simulink subsystem "Subsystem"  (R2025b)
settings: Solver=VariableStepAuto  StartTime=0.0  StopTime=10.0  RelTol=1e-3
values from neighbouring files (symbols this model uses):
  b2_ext = x(5)    [f_dynamics.m]    (also in f_dynamics_Wo_DT.m = 96.1986389127)
  b2_ret = x(6)    [f_dynamics.m]    (also in f_dynamics_Wo_DT.m = 15.072)
  Q = double(Q)    [EKF_delay_compensated.m]    (also in NO_DT_EKF_delay_compensated.m)
undefined symbols (not defined in the file or in its folder): P, T_S, x_0
libraries: simulink x1
settings Model: Creator=Mohamed Reda  LastModifiedBy=Mohamed Reda

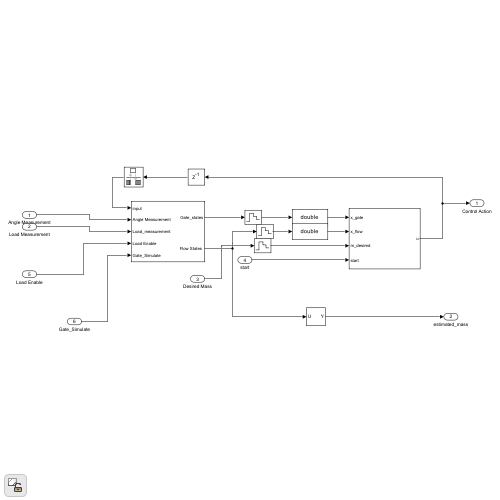
[thumbnail: Simulink's stored preview of the top-level diagram]
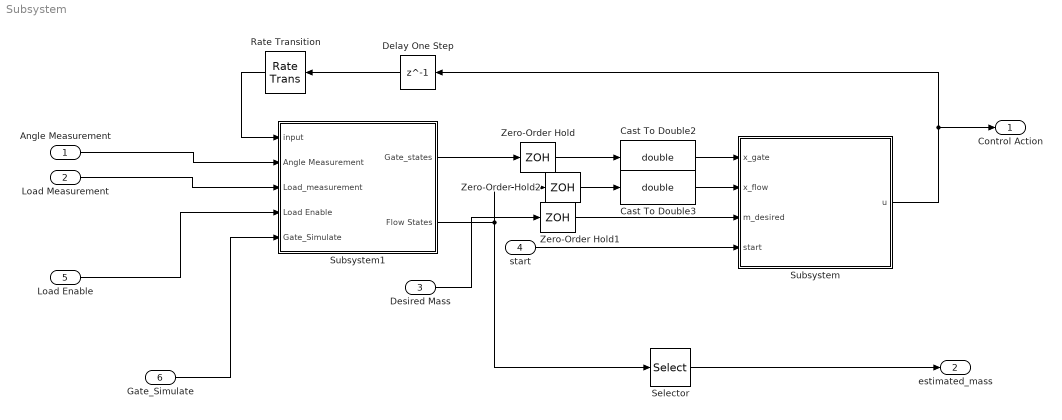
== system Subsystem ==
  Angle Measurement : Inport
  Load Measurement : Inport  Port=2
  Desired Mass : Inport  Port=3
  start : Inport  Port=4  SampleTime=5e-3
  Load Enable : Inport  Port=5
  Gate_Simulate : Inport  Port=6
  Cast To Double2 : DataTypeConversion  OutDataTypeStr=double  SaturateOnIntegerOverflow=off  RndMeth=Floor
  Cast To Double3 : DataTypeConversion  OutDataTypeStr=double  SaturateOnIntegerOverflow=off  RndMeth=Floor
  Delay One Step : Delay  DelayLength=1
  Rate Transition : RateTransition  OutPortSampleTime=2e-4
  Selector : Selector  InputPortWidth=9  IndexOptions=Index vector (dialog)  Indices=[2]  OutputSizes=1
  Subsystem : Subsystem
  Subsystem1 : Subsystem
  Zero-Order Hold : ZeroOrderHold  SampleTime=5e-3
  Zero-Order Hold1 : ZeroOrderHold  SampleTime=.5e-2
  Zero-Order Hold2 : ZeroOrderHold  SampleTime=5e-3
  Control Action : Outport
  estimated_mass : Outport  Port=2
  wires:
  Subsystem1/1(Gate_states) -> Zero-Order Hold/1
  Rate Transition/1 -> Subsystem1/1(input)
  Zero-Order Hold1/1 -> Subsystem/3(m_desired)
  Cast To Double3/1 -> Subsystem/2(x_flow)
  Delay One Step/1 -> Rate Transition/1
  Zero-Order Hold2/1 -> Cast To Double3/1
  Subsystem1/2("Flow States ") -> Selector/1, Zero-Order Hold2/1
  start/1 -> Subsystem/4(start)
  Cast To Double2/1 -> Subsystem/1(x_gate)
  Zero-Order Hold/1 -> Cast To Double2/1
  Selector/1 -> estimated_mass/1
  Subsystem/1(u) -> Control Action/1, Delay One Step/1
  Desired Mass/1 -> Zero-Order Hold1/1
  Angle Measurement/1 -> Subsystem1/2(Angle Measurement)
  Load Measurement/1 -> Subsystem1/3(Load_measurement)
  Load Enable/1 -> Subsystem1/4(Load Enable)
  Gate_Simulate/1 -> Subsystem1/5(Gate_Simulate)

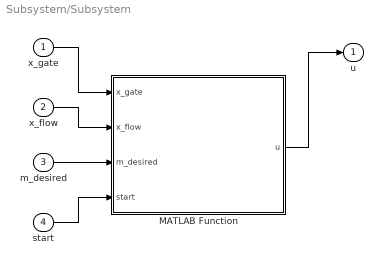
== system Subsystem/Subsystem ==
  x_gate : Inport  OutDataTypeStr=double  PortDimensions=7  SampleTime=[0.0050000000000000001,0]
  x_flow : Inport  Port=2  OutDataTypeStr=double  PortDimensions=9  SampleTime=[0.0050000000000000001,0]
  m_desired : Inport  Port=3  OutDataTypeStr=double  PortDimensions=1  SampleTime=[0.0050000000000000001,0]
  start : Inport  Port=4  OutDataTypeStr=double  PortDimensions=1  SampleTime=[0.0050000000000000001,0]
  MATLAB Function : MATLAB Function  TreatAsAtomicUnit=on
  u : Outport  OutDataTypeStr=double  PortDimensions=1  SampleTime=[0.0050000000000000001,0]
  wires:
  start/1 -> MATLAB Function/4(start)
  x_flow/1 -> MATLAB Function/2(x_flow)
  x_gate/1 -> MATLAB Function/1(x_gate)
  MATLAB Function/1(u) -> u/1
  m_desired/1 -> MATLAB Function/3(m_desired)

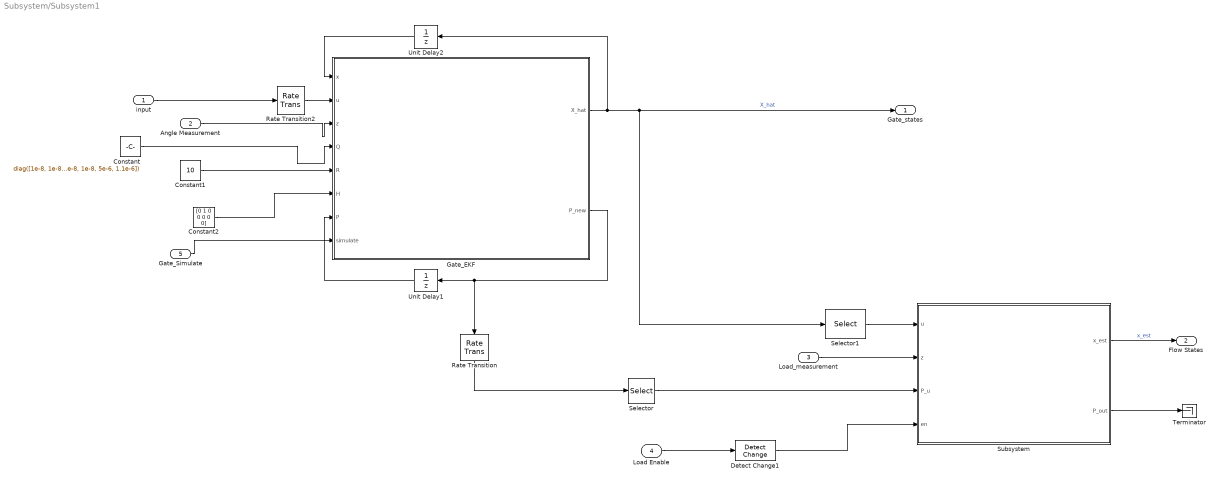
== system Subsystem/Subsystem1 ==
  input : Inport  OutDataTypeStr=double  PortDimensions=1  SampleTime=[0.00020000000000000001,0]
  Angle Measurement : Inport  Port=2  OutDataTypeStr=double  PortDimensions=1  SampleTime=[0.00020000000000000001,0]
  Load_measurement : Inport  Port=3  OutDataTypeStr=double  PortDimensions=1  SampleTime=[0.001,0]
  Load Enable : Inport  Port=4  OutDataTypeStr=boolean  PortDimensions=1  SampleTime=[0.001,0]
  Gate_Simulate : Inport  Port=5
  Constant : Constant  Value=diag([1e-8, 1e-8, 1e-8, 1e-8, 1e-8, 5e-6, 1.1e-6])
  Constant1 : Constant  Value=10
  Constant2 : Constant  Value=[0 1 0 0 0 0 0]
  Detect Change1 : simulink/Logic and Bit Operations/Detect Change  vinit=0  OutDataTypeStr=boolean
  Gate_EKF : MATLAB Function  TreatAsAtomicUnit=on
  Rate Transition : RateTransition
  Rate Transition2 : RateTransition
  Selector : Selector  NumberOfDimensions=2  InputPortWidth=7,7  IndexOptions=Index vector (dialog),Index vector (dialog)  Indices=1,1  OutputSizes=1,1
  Selector1 : Selector  InputPortWidth=7  IndexOptions=Index vector (dialog)  Indices=1  OutputSizes=1
  Subsystem : Subsystem
  Terminator : Terminator
  Unit Delay1 : UnitDelay  InitialCondition=diag([1e-6 1e-6 0.1 0.1 0.1 1e-6 1e-6])  SampleTime=-1  HasFrameUpgradeWarning=on
  Unit Delay2 : UnitDelay  InitialCondition=[deg2rad(0);0;9*101325;9*101325;101325;b2_ext;b2_ret]  SampleTime=-1  HasFrameUpgradeWarning=on
  Gate_states : Outport  OutDataTypeStr=double  PortDimensions=7  SampleTime=[0.00020000000000000001,0]
  "Flow States " : Outport  Port=2  OutDataTypeStr=double  PortDimensions=9  SampleTime=[0.001,0]
  wires:
  Gate_Simulate/1 -> Gate_EKF/8(simulate)
  Constant/1 -> Gate_EKF/4(Q)
  Selector/1 -> Subsystem/3(P_u)
  Load_measurement/1 -> Subsystem/2(z)
  Gate_EKF/1(X_hat) -> Unit Delay2/1, Selector1/1, Gate_states/1  "X_hat"
  input/1 -> Rate Transition2/1
  Subsystem/2(P_out) -> Terminator/1
  Detect Change1/1 -> Subsystem/4(en)
  Load Enable/1 -> Detect Change1/1
  Rate Transition/1 -> Selector/1
  Selector1/1 -> Subsystem/1(u)
  Unit Delay1/1 -> Gate_EKF/7(P)
  Angle Measurement/1 -> Gate_EKF/3(z)
  Gate_EKF/2(P_new) -> Rate Transition/1, Unit Delay1/1
  Unit Delay2/1 -> Gate_EKF/1(x)
  Rate Transition2/1 -> Gate_EKF/2(u)
  Subsystem/1(x_est) -> "Flow States "/1  "x_est"
  Constant2/1 -> Gate_EKF/6(H)
  Constant1/1 -> Gate_EKF/5(R)

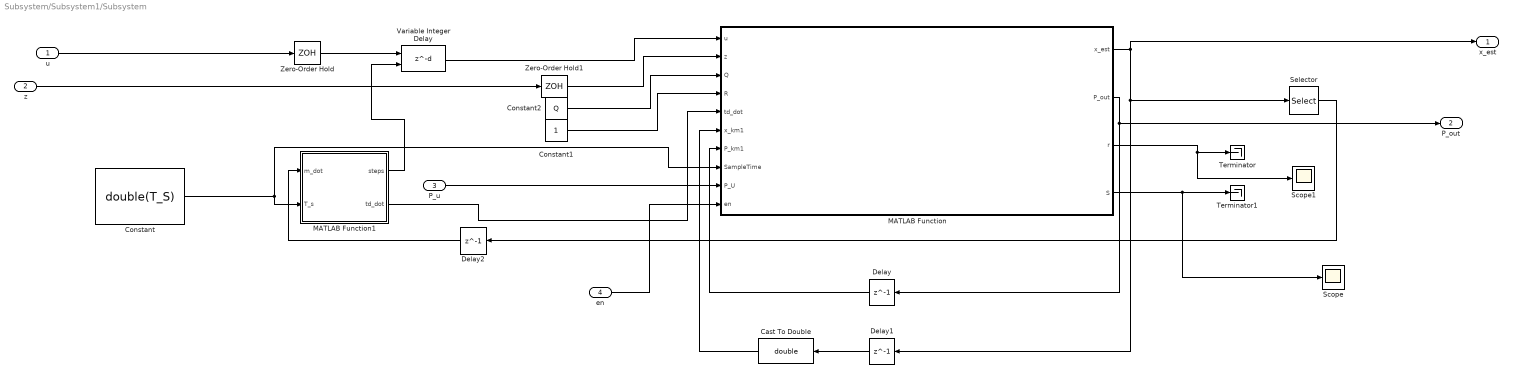
== system Subsystem/Subsystem1/Subsystem ==
  u : Inport
  z : Inport  Port=2
  P_u : Inport  Port=3
  en : Inport  Port=4
  Cast To Double : DataTypeConversion  OutDataTypeStr=double  SaturateOnIntegerOverflow=off  RndMeth=Floor
  Constant : Constant  Value=double(T_S)  OutDataTypeStr=double
  Constant1 : Constant
  Constant2 : Constant  Value=Q
  Delay : Delay  DelayLength=1  InitialCondition=P  SampleTime=T_S
  Delay1 : Delay  DelayLength=1  InitialCondition=x_0  SampleTime=T_S
  Delay2 : Delay  DelayLength=1  InputProcessing=Columns as channels (frame based)
  MATLAB Function : MATLAB Function  TreatAsAtomicUnit=on
  MATLAB Function1 : MATLAB Function  TreatAsAtomicUnit=on
  Scope : Scope
  Scope1 : Scope
  Selector : Selector  InputPortWidth=9  IndexOptions=Index vector (dialog)  Indices=1  OutputSizes=1
  Terminator : Terminator
  Terminator1 : Terminator
  Variable Integer Delay : Delay  DelayLengthSource=Input port  DelayLengthUpperLimit=500
      settings: InputPortMap=u0,p1
  Zero-Order Hold : ZeroOrderHold  SampleTime=T_S
  Zero-Order Hold1 : ZeroOrderHold  SampleTime=T_S
  x_est : Outport  OutDataTypeStr=double
  P_out : Outport  Port=2
  wires:
  Constant/1 -> MATLAB Function1/2(T_s), MATLAB Function/8(SampleTime)
  Delay/1 -> MATLAB Function/7(P_km1)
  MATLAB Function/2(P_out) -> Delay/1, P_out/1
  Constant1/1 -> MATLAB Function/4(R)
  Cast To Double/1 -> MATLAB Function/6(x_km1)
  P_u/1 -> MATLAB Function/9(P_U)
  Zero-Order Hold/1 -> Variable Integer Delay/1
  MATLAB Function1/1(steps) -> Variable Integer Delay/2
  MATLAB Function/4(S) -> Scope/1, Terminator1/1
  u/1 -> Zero-Order Hold/1
  MATLAB Function/3(r) -> Scope1/1, Terminator/1
  Variable Integer Delay/1 -> MATLAB Function/1(u)
  z/1 -> Zero-Order Hold1/1
  MATLAB Function/1(x_est) -> Delay1/1, Selector/1, x_est/1
  Zero-Order Hold1/1 -> MATLAB Function/2(z)
  Selector/1 -> Delay2/1
  Delay2/1 -> MATLAB Function1/1(m_dot)
  MATLAB Function1/2(td_dot) -> MATLAB Function/5(td_dot)
  Delay1/1 -> Cast To Double/1
  en/1 -> MATLAB Function/10(en)
  Constant2/1 -> MATLAB Function/3(Q)

== matlab function Subsystem/Subsystem1/Gate_EKF ==
  settings: updateMethod=DISCRETE  sampleTime=2e-4
  data: x input; u input; X_hat output; P_new output size=[7 7]; z input; Q input; R input; H input; P input; simulate input
function [X_hat,P_new] = EKF(x,u,z,Q,R,H,P,simulate)
persistent first_run 
if isempty(first_run)
    first_run = 1;
    P(6,6) = 1e-8;
    P(7,7) = 1e-8;

end
%% prediction
    x_prior=x;
    for i=1:10
    x_prior = f_dynamics(x_prior,u,2e-5);
    end
    J = Jacobian(x,u,2e-4);
    if(simulate)
        X_hat = x_prior;
        P_new = zeros(7,7);
        return
    end
    P_prior = J * P * J' + Q;

%% innovation
    r = (z - H' * x_prior);
    S = (H'*P_prior*H+R);
    K = P_prior * H / S;
%% update
    %I=eye(7);
    %I_KH=I-K*H';
    P_new = P_prior - K * H' * P_prior;
    X_hat = x_prior + K * r;
end

== matlab function Subsystem/Subsystem1/Subsystem/MATLAB Function ==
  settings: updateMethod=DISCRETE  sampleTime=T_S
  data: u input; x_est output double; z input; Q input; R input; td_dot input; x_km1 input; P_km1 input; SampleTime input; P_out output; r output; S output; P_U input; en input
function [x_est,P_out,r,S] = EKF(u,z,Q,R,td_dot,x_km1,P_km1,SampleTime,P_U,en)
[x_est,P_out,r,S] = EKF_delay_compensated(u,z,Q,R,td_dot,x_km1,P_km1,SampleTime,P_U,en);
end

== matlab function Subsystem/Subsystem1/Subsystem/MATLAB Function1 ==
  settings: updateMethod=DISCRETE  sampleTime=T_S
  data: m_dot input double; steps output int16; T_s input double; td_dot output double
function [steps, td_dot] = delay_steps(m_dot,T_s)
if m_dot>1e-3
    tk=0.162;
else
    tk=0.401;
end
[td, td_dot] = Transport_time(tk,T_s);
steps=int16(td/T_s);
end

== matlab function Subsystem/MATLAB Function ==
  data: x_gate input; u output; x_flow input; m_desired input; start input
function u  = MPC(x_gate,x_flow,m_desired,start)
u=0;
[u] = NMPC(x_gate,x_flow,m_desired,start);
